simulink model "RadarSimulinkProjectRev011"  (R2024a)
settings: Solver=VariableStepAuto  StartTime=0.0  StopTime=0.0125*2  RelTol=1e-3
values from neighbouring files (symbols this model uses):
  AngleTime = SweepTime/10    (= 10000)    [InitializationOfVariablesRev000.m]    (also in InitializationOfVariablesRev001.m; InitializationOfVariablesRev002.m = 2000; InitializationOfVariablesRev003.m = 20000; InitializationOfVariablesRev004.m = 2097152)
  ASR_LUT = Rsamp    [InitializationOfVariablesRev003.m]    (also in InitializationOfVariablesRev004.m = round((R*2*SystemFs)/c); InitializationOfVariablesRev005.m = round((R*2*SystemFs)/c))
  Btn_Debounce = 20000    [InitializationOfVariablesRev003.m]    (also in InitializationOfVariablesRev004.m; InitializationOfVariablesRev005.m)
  ChirpNc = 128    [InitializationOfVariablesRev004.m]    (also in InitializationOfVariablesRev005.m)
  ChirpSizeLength = length(FCW)    [InitializationOfVariablesRev004.m]    (also in InitializationOfVariablesRev005.m = 16384)
  DeciFactor = 8    [InitializationOfVariablesRev005.m]
  FCW = [FCW_p1, FCW_p2]    [InitializationOfVariablesRev002.m]    (also in InitializationOfVariablesRev003.m; InitializationOfVariablesRev004.m = interp1(1:length(FCW_base), FCW_base,      linspace(1, lengt; InitializationOfVariablesRev005.m = f / SystemFs)
  RXFFTLength = 4096    [InitializationOfVariablesRev003.m]    (also in InitializationOfVariablesRev004.m = 1024; InitializationOfVariablesRev005.m = 2048)
  SweepTime = 100000    [InitializationOfVariablesRev000.m]    (also in InitializationOfVariablesRev001.m; InitializationOfVariablesRev002.m = 20000; InitializationOfVariablesRev003.m = 200000; InitializationOfVariablesRev004.m = 23068672)
undefined symbols (not defined in the file or in its folder): SignalGenerationForAnalysis, Subsystem, xc7a200tfbg676
libraries: hdlBasic x453, hdlUtilities x11, hdlDSPIP x11, vmcUtilities x1
(part 5 of 5)

== system RadarSimulinkProjectRev011/RangeProcessing/Subsystem ==
  note: For radix burst, tlast should come from each chirp end,
      | in this case, tlast triggers every 128 samples, (0, 2048, 4096..ect until 262,000th data point, then moves on to the next set at 1, 2049, 4097, ect.)
  note: Chirp*FFT=total data
      | 128*2048=262,000
  note: Needs to be 0, 1024, 2048
      | Then 1, 1025, 2049, ect
  tvalid : Inport
  Reset : Inport  Port=2
  Chirp : hdlBasic/Counter  cnt_type=Count limited  cnt_to=ChirpNc-1  operation=Up  start_count=0  cnt_by_val=1  arith_type=Unsigned  n_bits=8  bin_pt=0  load_pin=off  rst=on  en=on  explicit_period=Explicit  period=P1  use_behavioral_HDL=off  implementation=Fabric  XmcBlockStatus=1  maskContainerNames=group1  block_type=counter  block_config=sysgen:Counter_config  block_width=531  block_height=1023
  Constant : hdlBasic/Constant  const=ChirpNc-1  gui_display_data_type=Fixed-point  arith_type=Signed (2's comp)  n_bits=16  bin_pt=0  preci_type=Single  exp_width=8  frac_width=24  explicit_period=off  period=1  XmcBlockStatus=1  maskContainerNames=tabcontainer1  block_type=constant  block_config=sysgen:Constant_config
  Constant1 : hdlBasic/Constant  const=RXFFTLength  gui_display_data_type=Fixed-point  arith_type=Signed (2's comp)  n_bits=16  bin_pt=0  preci_type=Single  exp_width=8  frac_width=24  explicit_period=off  period=1  XmcBlockStatus=1  maskContainerNames=tabcontainer1  block_type=constant  block_config=sysgen:Constant_config
  FFT : hdlBasic/Counter  cnt_type=Count limited  cnt_to=RXFFTLength-1  operation=Up  start_count=0  cnt_by_val=1  arith_type=Unsigned  n_bits=13  bin_pt=0  load_pin=off  rst=on  en=on  explicit_period=Explicit  period=P1  use_behavioral_HDL=off  implementation=Fabric  XmcBlockStatus=1  maskContainerNames=group1  block_type=counter  block_config=sysgen:Counter_config  block_width=531  block_height=1023
  MultAdd : hdlBasic/MultAdd  mode=Addition  en=off  latency=0  precision=User Defined  arith_type=Unsigned  n_bits=18  bin_pt=0  XmcBlockStatus=1  maskContainerNames=tabcontainer1  block_type=multadd  block_config=sysgen:MultAdd_config
  Relational : hdlBasic/Relational  mode=a=b  op_type=Bool  en=off  latency=0  XmcBlockStatus=1  maskContainerNames=tabcontainer1  block_type=relational  block_config=sysgen:Relational_config
  AddrOut : Outport
  FFTtlast : Outport  Port=2
  wires:
  Reset/1 -> FFT/1, Chirp/1
  tvalid/1 -> Chirp/2
  Chirp/1 -> MultAdd/1, Relational/1
  Constant/1 -> Relational/2
  Relational/1 -> FFTtlast/1, FFT/2
  Constant1/1 -> MultAdd/2
  FFT/1 -> MultAdd/3
  MultAdd/1 -> AddrOut/1

== system RadarSimulinkProjectRev011/Velocity Processing/FFTTracking ==
  note: Should restart counter at beggining or end,
      | In Radix mode, Tlast is not the beggining because there is a gap
  note: In Radix burst, this is active for only real frame of data
      | In Pipeline, it's always active
  note: Bring back to 0 at start
  data_Active : Inport
  StatusReady : Inport  Port=2
  Delay : hdlBasic/Delay  rst=off  en=off  latency=4  reg_retiming=off  XmcBlockStatus=1  maskContainerNames=group1  block_type=delay  block_config=sysgen:Delay_config
  IndexTracker : hdlBasic/Counter  cnt_type=Count limited  cnt_to=ChirpNc-1  operation=Up  start_count=0  cnt_by_val=1  arith_type=Unsigned  n_bits=14  bin_pt=0  load_pin=off  rst=on  en=on  explicit_period=Explicit  period=P1  use_behavioral_HDL=off  implementation=Fabric  XmcBlockStatus=1  maskContainerNames=group1  block_type=counter  block_config=sysgen:Counter_config  block_width=531  block_height=1023
  Inverter : hdlBasic/Inverter  en=off  latency=0  XmcBlockStatus=1  maskContainerNames=group2  block_type=inv  block_config=sysgen:Inverter_config
  Logical1 : hdlBasic/Logical  logical_function=AND  inputs=2  en=off  latency=0  precision=Full  arith_type=Unsigned  n_bits=16  bin_pt=0  align_bp=on  overflow=[]  quantization=[]  XmcBlockStatus=1  maskContainerNames=tabcontainer1  block_type=logical  block_config=sysgen:Logical_config
  FFTIndex : Outport
  PeakSerachEnable : Outport  Port=2
  wires:
  IndexTracker/1 -> FFTIndex/1
  Inverter/1 -> IndexTracker/1
  Logical1/1 -> Delay/1
  StatusReady/1 -> Logical1/1, Inverter/1
  data_Active/1 -> Logical1/2
  Delay/1 -> PeakSerachEnable/1, IndexTracker/2

== system RadarSimulinkProjectRev011/Velocity Processing/Peak Detection ==
  note: Tlast needs to arrive after data has propagated to register
  note: Is previous sample more than stored?
  Tlast : Inport
  FFTInput : Inport  Port=2
  FFTIndexTrack : Inport  Port=3
  FFTValidMask : Inport  Port=4
  Mux : hdlBasic/Mux  inputs=2  en=off  latency=0  precision=Full  arith_type=Unsigned  n_bits=16  bin_pt=14  quantization=Truncate  overflow=Wrap  XmcBlockStatus=1  maskContainerNames=tabcontainer1  block_type=mux  block_config=sysgen:Mux_config
  Mux1 : hdlBasic/Mux  inputs=2  en=off  latency=0  precision=Full  arith_type=Unsigned  n_bits=16  bin_pt=14  quantization=Truncate  overflow=Wrap  XmcBlockStatus=1  maskContainerNames=tabcontainer1  block_type=mux  block_config=sysgen:Mux_config
  Prev1 : hdlBasic/Delay  rst=off  en=off  latency=5  reg_retiming=off  XmcBlockStatus=1  maskContainerNames=group1  block_type=delay  block_config=sysgen:Delay_config
  Prev2 : hdlBasic/Delay  rst=off  en=off  latency=4  reg_retiming=off  XmcBlockStatus=1  maskContainerNames=group1  block_type=delay  block_config=sysgen:Delay_config
  Register : hdlBasic/Register  init=0  rst=on  en=off  XmcBlockStatus=1  maskContainerNames=tabcontainer1  block_type=register  block_config=sysgen:Register_config
  Register1 : hdlBasic/Register  init=0  rst=on  en=off  XmcBlockStatus=1  maskContainerNames=tabcontainer1  block_type=register  block_config=sysgen:Register_config
  Relational : hdlBasic/Relational  mode=a>b  op_type=Bool  en=on  latency=1  XmcBlockStatus=1  maskContainerNames=tabcontainer1  block_type=relational  block_config=sysgen:Relational_config
  WriteEnable : Outport
  DataMag : Outport  Port=2
  DataINDX : Outport  Port=3
  PeakFound : Outport  Port=4
  Tlast_delayed : Outport  Port=5
  wires:
  FFTValidMask/1 -> Relational/3
  FFTInput/1 -> Mux/3, Relational/1
  Register/1 -> Relational/2, DataMag/1, Mux/2
  Mux/1 -> Register/1
  Register1/1 -> DataINDX/1, Mux1/2
  FFTIndexTrack/1 -> Mux1/3
  Mux1/1 -> Register1/1
  Prev1/1 -> Register1/2, Register/2, Tlast_delayed/1
  Relational/1 -> Mux1/1, Mux/1, PeakFound/1
  Tlast/1 -> Prev2/1, Prev1/1
  Prev2/1 -> WriteEnable/1

== system RadarSimulinkProjectRev011/Velocity Processing/Peak Detection1 ==
  note: Tlast needs to arrive after data has propagated to register
  note: Is previous sample more than stored?
  Tlast : Inport
  FFTInput : Inport  Port=2
  FFTIndexTrack : Inport  Port=3
  FFTValidMask : Inport  Port=4
  Mux : hdlBasic/Mux  inputs=2  en=off  latency=0  precision=Full  arith_type=Unsigned  n_bits=16  bin_pt=14  quantization=Truncate  overflow=Wrap  XmcBlockStatus=1  maskContainerNames=tabcontainer1  block_type=mux  block_config=sysgen:Mux_config
  Mux1 : hdlBasic/Mux  inputs=2  en=off  latency=0  precision=Full  arith_type=Unsigned  n_bits=16  bin_pt=14  quantization=Truncate  overflow=Wrap  XmcBlockStatus=1  maskContainerNames=tabcontainer1  block_type=mux  block_config=sysgen:Mux_config
  Prev1 : hdlBasic/Delay  rst=off  en=off  latency=5  reg_retiming=off  XmcBlockStatus=1  maskContainerNames=group1  block_type=delay  block_config=sysgen:Delay_config
  Prev2 : hdlBasic/Delay  rst=off  en=off  latency=4  reg_retiming=off  XmcBlockStatus=1  maskContainerNames=group1  block_type=delay  block_config=sysgen:Delay_config
  Register : hdlBasic/Register  init=0  rst=on  en=off  XmcBlockStatus=1  maskContainerNames=tabcontainer1  block_type=register  block_config=sysgen:Register_config
  Register1 : hdlBasic/Register  init=0  rst=on  en=off  XmcBlockStatus=1  maskContainerNames=tabcontainer1  block_type=register  block_config=sysgen:Register_config
  Relational : hdlBasic/Relational  mode=a>b  op_type=Bool  en=on  latency=1  XmcBlockStatus=1  maskContainerNames=tabcontainer1  block_type=relational  block_config=sysgen:Relational_config
  WriteEnable : Outport
  DataMag : Outport  Port=2
  DataINDX : Outport  Port=3
  PeakFound : Outport  Port=4
  Tlast_delayed : Outport  Port=5
  wires:
  FFTValidMask/1 -> Relational/3
  Tlast/1 -> Prev1/1, Prev2/1
  Register/1 -> Relational/2, DataMag/1, Mux/2
  Mux/1 -> Register/1
  Register1/1 -> DataINDX/1, Mux1/2
  FFTIndexTrack/1 -> Mux1/3
  Mux1/1 -> Register1/1
  Prev1/1 -> Register1/2, Register/2, Tlast_delayed/1
  FFTInput/1 -> Relational/1, Mux/3
  Relational/1 -> Mux1/1, Mux/1, PeakFound/1
  Prev2/1 -> WriteEnable/1

== matlab function RadarSimulinkProjectRev011/MATLAB Function ==
  data: a input; b input; c input; d input; ao output; noisePower input; bo output; co output; do output
function [ao,bo,co,do] = fcn(a,b,c,d,noisePower)
    noise = noisePower*randn(size(a));
    ao = real(a)+noise;
    bo = real(b)+noise;
    co = real(c)+noise;
    do = real(d)+noise;
end
